simulink model "Angular_Transformation_Matrix"  (R2018a)
settings: Solver=VariableStepAuto  StartTime=0.0  StopTime=10.0  RelTol=1e-3
libraries: simulink_extras x2
settings Model: Creator=Ibrahim  LastModifiedBy=Ibrahim

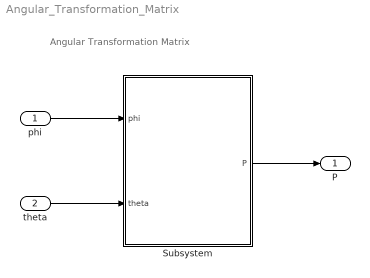
== system Angular_Transformation_Matrix ==
  note: Angular Transformation Matrix
  phi : Inport
  theta : Inport  Port=2
  Subsystem : Subsystem
  P : Outport
  wires:
  phi/1 -> Subsystem/1(phi)
  theta/1 -> Subsystem/2(theta)
  Subsystem/1(P) -> P/1

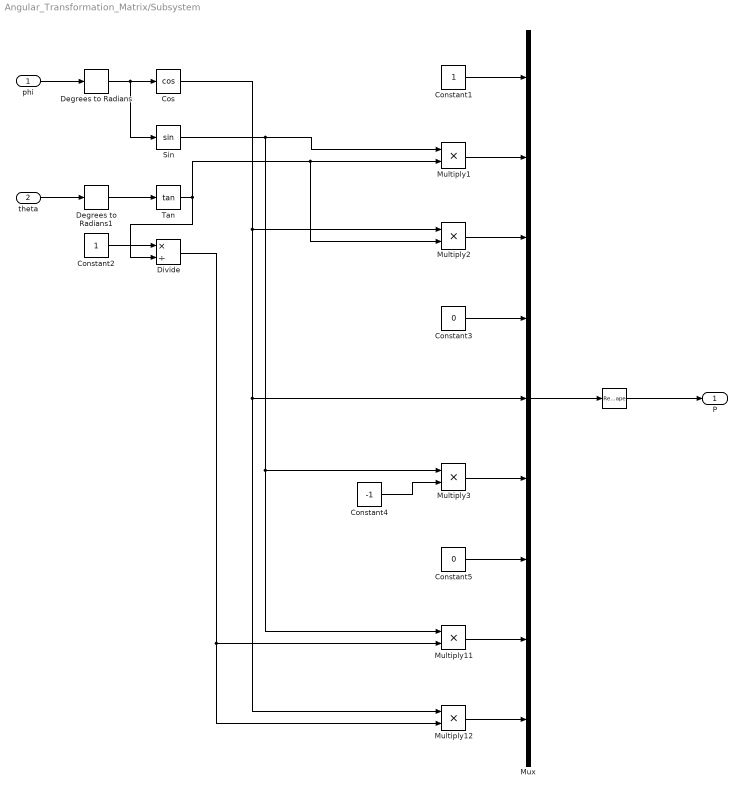
== system Angular_Transformation_Matrix/Subsystem ==
  phi : Inport
  theta : Inport  Port=2
  " " : Reshape  OutputDimensionality=Customize  OutputDimensions=[3,3]
  Constant1 : Constant
  Constant2 : Constant
  Constant3 : Constant  Value=0
  Constant4 : Constant  Value=-1
  Constant5 : Constant  Value=0
  Cos : Trigonometry  Operator=cos
  Degrees to Radians : simulink_extras/Transformations/Degrees to Radians
  Degrees to Radians1 : simulink_extras/Transformations/Degrees to Radians
  Divide : Product  Inputs=*/
  Multiply{1..3,11..12} (5 alike) : Product
  Mux : Mux  Inputs=9
  Sin : Trigonometry
  Tan : Trigonometry  Operator=tan
  P : Outport
  wires:
  Mux/1 -> " "/1
  Degrees to Radians/1 -> Cos/1, Sin/1
  Tan/1 -> Multiply2/2, Multiply1/2, Divide/2
  Constant1/1 -> Mux/1
  Sin/1 -> Multiply11/1, Multiply3/1, Multiply1/1
  Cos/1 -> Multiply12/1, Mux/5, Multiply2/1
  Constant4/1 -> Multiply3/2
  Multiply11/1 -> Mux/8
  Multiply12/1 -> Mux/9
  Degrees to Radians1/1 -> Tan/1
  Divide/1 -> Multiply12/2, Multiply11/2
  Constant5/1 -> Mux/7
  Multiply3/1 -> Mux/6
  Constant2/1 -> Divide/1
  Multiply1/1 -> Mux/2
  Multiply2/1 -> Mux/3
  Constant3/1 -> Mux/4
  " "/1 -> P/1
  phi/1 -> Degrees to Radians/1
  theta/1 -> Degrees to Radians1/1
